simulink model "MODOSDESLISANTES"  (R2025a)
settings: Solver=VariableStepAuto  StartTime=0.0  StopTime=10.0  RelTol=1e-3
InitFcn:
  | % --- Código para el InitFcn ---
  | 
  | % Añadir la API al path (asegúrate que la ruta es correcta)
  | addpath('C:/RoboDK/Matlab/');
  | 
  | % Declarar las variables como globales
  | global RDK;
  | global ROBOT;
  | 
  | % Iniciar la conexión
  | RDK = Robolink();
  | 
  | % Obtener tu robot (CAMBIA 'MiRobot' por el nombre de tu robot)
  | ROBOT = RDK.Item('Fanuc CRX-5iA', RDK.ITEM_TYPE_ROBOT);
  | 
  | % Fallar si no se encuentra
  | if ~ROBOT.Valid()
  |     error('No se encontró el robot "MiRobot" en RoboDK.');
  | end
  | 
  | % Ajustar el modo de ejecución a SIMULATE
  | % Esto es necesario para que el streaming funcione bien.
  | RDK.setRunMode(RDK.RUNMODE_SIMULATE);
  | 
  | % Mover a una posición inicial de forma segura (opcional)
  | % ROBOT.MoveJ([0, -90, 0, -90, 0, 0]);
  | 
  | fprintf('RoboDK Conectado y listo para Simulink.\n');
  | % --- Fin del código InitFcn ---
libraries: robotmaniplib x1, robotsim3dlib x1, sim3dlib x1
settings Model: Creator=Sandro  LastModifiedBy=jaros

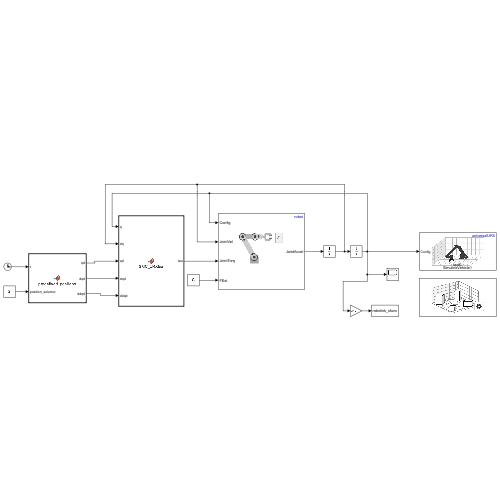
[thumbnail: Simulink's stored preview of the top-level diagram]
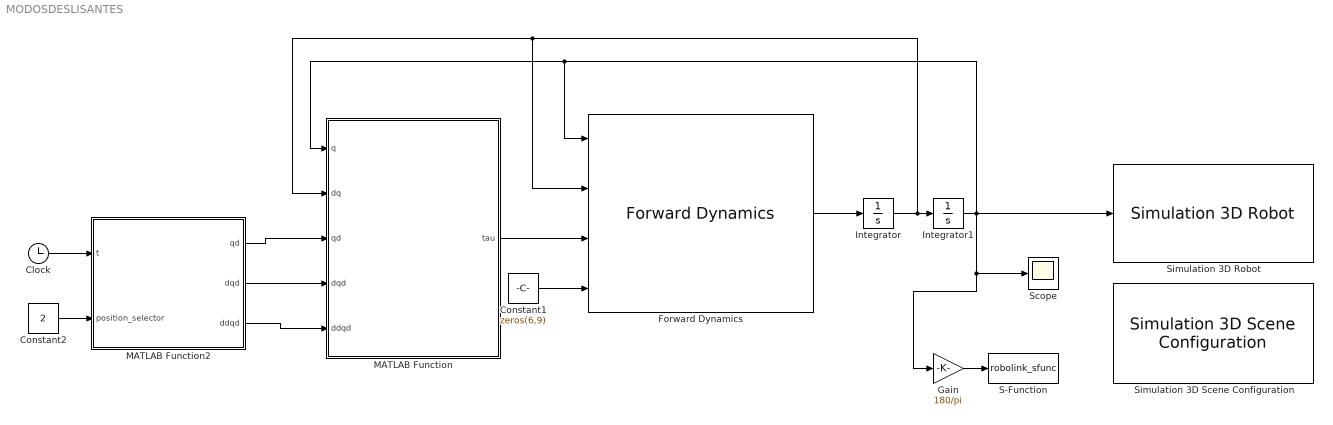
== system MODOSDESLISANTES ==
  Clock : Clock
  Constant1 : Constant  Value=zeros(6,9)
  Constant2 : Constant  Value=2
  Forward Dynamics : robotmaniplib/Forward Dynamics  RigidBodyTree=robot  SimulateUsing=Interpreted execution
  Gain : Gain  Gain=180/pi
  Integrator : Integrator
  Integrator1 : Integrator
  MATLAB Function : MATLAB Function  TreatAsAtomicUnit=on
  MATLAB Function2 : MATLAB Function  TreatAsAtomicUnit=on
  S-Function : S-Function  FunctionName=robolink_sfunc  SFunctionDeploymentMode=off  EnableBusSupport=off
  Scope : Scope
      settings: ActiveDisplayYMinimum=-2.2920470926945278  ActiveDisplayYMaximum=1.7511974378235475
  Simulation 3D Robot : robotsim3dlib/Simulation 3D Robot  actorInputType=Robot Library  RigidBodyTree=universalUR5  ActorName=SimulinkVehicle1  existActorChekBox=off  initialTrans=[0 0 0]  initialRot=[0 0 0]  initialConfig="[0  0  0  0  0  0]"  EndEffector=tool0  eeOffsetInpChekBox=off  eeTargetTrans=[0 0 0]  eeTargetRot=[0 0 0]  enableRegionGraspChekBox=off  regionGraspInpChekBox=off  eeTargTransDiff=[0.2 0.2 0.2]  eeTargRotDiff=[0 0 0]  enableVisualVisualization=on  enableCollisionVisualization=off  collisionGeomColor=[0 1 0]  collisionGeomTransp=0.1  inpConfEnbVal=on  inpGraspEnbVal=off  inpTransEnbVal=off  outConfEnbVal=off  outGraspEnbVal=off  outTransEnbVal=off  SampleTime=0.01  ActorType=SimulinkVehicle  ID=1  aMode=6  ActorTag=SimulinkVehicle1  Mesh=RigidBodyTree
  Simulation 3D Scene Configuration : sim3dlib/Simulation 3D Scene Configuration  Priority=0  ProjectFormat=Default Scenes  SceneDesc=Empty scene  ProjectName=C:\Program Files\MATLAB\R2025a\toolbox\shared\sim3d_projects\automotive_project_windows\UE\WindowsNoEditor\VehicleSimulation.exe  ScenePath=/Game/Maps/EmptyScene  EnableOpenDRIVE=off  vehTagList={'<empty>';'Custom';'Scene Origin';'SimulinkVehicle1'}  vehTag=Scene Origin  AttachedCameraRelativeTranslation=[0 0 0]  FreeCameraDefaultInitialTranslation=[-6, 0, 2]  AttachedCameraRelativeRotation=[0 0 0]  FreeCameraDefaultInitialRotation=[0, -15, 0]  ViewpointName=Custom  FreeCameraInitialTranslation=[0 0 0]  ViewpointTranslation=[0 0 0]  FreeCameraInitialRotation=[0 0 0]  ViewpointRotation=[0 0 0]  OpVisEn=off  Ts=0.02  EnableWindow=on  EnableRemoteAccess=off  EnableWeather=off  SunAzimuth=90  SunAltitude=40.0  EnableGeospatialSun=off  Latitude=0  Longitude=0  Date=2023-01-01  Time=10:30:00  GeoTimeZone=-5.0  SunDaylightSaving=off  wind=1  clouds=10  EnableVolumetricClouds=off  CloudCoverage=0  CloudAltitude=6  fog=0  rain=0  RaindropsEffect=off  SnowDensity=0  EnableGeospatial=off  TilesetSource=Earth terrain  UseTrueOrigin=off  OriginHeight=200  OriginLatitude=40.744652  OriginLongitude=-73.988864  MapStyle=Aerial  AdditionalAssetIDs=[]  UseAdvancedSunSky=off  SolarTime=11  TimeZone=-5  Day=21  Month=9  Year=2022  UseDaylightSavingTime=on  DSTStartDay=10  DSTStartMonth=3  DSTEndDay=3  DSTEndMonth=11  DSTSwitchHour=2  sensorTag=MainCamera1  sensorId=1  sensorName=MainCamera1  mountLoc=Origin  offsetFlag=off  tmountOffset=[0, 0, 0]  rmountOffset=[0, 0, 0]  HorizontalResolution=1280  VerticalResolution=720  HorizontalFOV=60  mountPoint=[0 0 0]  mountOrientation=[0 0 0]  aMode=6  ID=1  GeoTrigger=Inactive  ViewNameList={'Custom'}  ViewTranslationList={'[0 0 0]'}  ViewRotationList={'[0 0 0]'}
      settings: LibrarySourceBlock=robotsim3dlib/Simulation 3D Scene Configuration
  wires:
  Forward Dynamics/1 -> Integrator/1
  Integrator/1 -> MATLAB Function/2(dq), Forward Dynamics/2, Integrator1/1
  Integrator1/1 -> Simulation 3D Robot/1, Scope/1, Gain/1, Forward Dynamics/1, MATLAB Function/1(q)
  Constant1/1 -> Forward Dynamics/4
  MATLAB Function2/2(dqd) -> MATLAB Function/4(dqd)
  Constant2/1 -> MATLAB Function2/2(position_selector)
  MATLAB Function2/3(ddqd) -> MATLAB Function/5(ddqd)
  Clock/1 -> MATLAB Function2/1(t)
  MATLAB Function2/1(qd) -> MATLAB Function/3(qd)
  MATLAB Function/1(tau) -> Forward Dynamics/3
  Gain/1 -> S-Function/1

== matlab function MODOSDESLISANTES/MATLAB Function ==
  data: q input; dq input; tau output; qd input; dqd input; ddqd input
function tau = SMC_CRX5ia(q, dq, qd, dqd, ddqd)
% Control por Modos Deslizantes para Fanuc CRX-5ia
% Parámetros definidos internamente - Sin estructura
%
% Inputs:
%   q, dq      : Estados actuales [6x1] (rad, rad/s)
%   qd, dqd, ddqd: Trayectoria deseada [6x1]
%
% Output:
%   tau        : Vector de torque [6x1] (Nm)

%#codegen
tau = zeros(6,1); % Especificar tamaño de salida

% =========================================================================
% PARÁMETROS DEFINIDOS INTERNAMENTE (Basados en URDF del CRX-5ia)
% =========================================================================

% 1. MATRIZ DE INERCIA ESTIMADA [kg·m²]
M_hat = diag([2.5, 1.8, 1.2, 0.8, 0.5, 0.3]);

% 2. MATRIZ DE CORIOLIS ESTIMADA
C_hat = zeros(6,6); % Simplificación inicial

% 3. VECTOR DE GRAVEDAD [Nm]
g_hat = [0; 12.5; 8.8; 0; 2.9; 0.3];

% 4. MATRIZ DE GANANCIAS DE SUPERFICIE DESLIZANTE
Lambda = diag([8, 8, 10, 12, 15, 15]);

% 5. MATRIZ DE GANANCIAS DISCONTINUAS
K = diag([25, 20, 15, 10, 8, 5]);

% 6. PARÁMETRO DE ROBUSTEZ
eta = 3;

% 7. CONFIGURACIÓN ANTI-CHATTERING
use_saturation = true;
phi = 0.15;

% 8. LÍMITES ARTICULARES (del URDF)
q_min = [-2*pi, -2*pi, -pi, -2*pi, -2*pi, -2*pi]';
q_max = [2*pi, 2*pi, pi, 2*pi, 2*pi, 2*pi]';
dq_max = [3.15, 3.15, 3.15, 3.2, 3.2, 3.2]';

% =========================================================================
% ALGORITMO DE CONTROL POR MODOS DESLIZANTES
% =========================================================================

% Verificación de límites articulares
q = clamp(q, q_min, q_max);
dq = clamp(dq, -dq_max, dq_max);

% Cálculo de errores
q_tilde = q - qd;
dq_tilde = dq - dqd;

% Velocidad y aceleración de referencia
dq_r = dqd - Lambda * q_tilde;
ddq_r = ddqd - Lambda * dq_tilde;

% Superficie deslizante
s = dq - dq_r;

% Control equivalente
tau_eq = M_hat * ddq_r + C_hat * dq_r + g_hat;

% Término robusto (con saturación para reducir chattering)
if use_saturation
    s_robust = saturation(s, phi);
else
    s_robust = sign(s);
end

% Ley de control final
tau = tau_eq - K * s_robust - eta * s;

% Limitar torque de salida para protección
tau_max = [100, 80, 60, 40, 30, 20]'; % [Nm] límites conservadores
tau = clamp(tau, -tau_max, tau_max);

end

% =========================================================================
% FUNCIONES AUXILIARES
% =========================================================================

function s_sat = saturation(s, phi)
% Función de saturación para reducir chattering
    s_sat = zeros(size(s));
    for i = 1:length(s)
        if abs(s(i)) > phi
            s_sat(i) = sign(s(i));
        else
            s_sat(i) = s(i) / phi;
        end
    end
end

function y = clamp(x, min_val, max_val)
% Función de limitación de valores
    y = min(max(x, min_val), max_val);
end

== matlab function MODOSDESLISANTES/MATLAB Function2 ==
  data: qd output; t input; position_selector input; dqd output; ddqd output
function [qd, dqd, ddqd] = predefined_positions(t, position_selector)
% Posiciones predefinidas para el CRX-5ia
%
% position_selector:
%   1: Home (todo ceros)
%   2: Configuración extendida
%   3: Configuración recogida
%   4: Posición de trabajo
%   5: Personalizada (puedes agregar más)

    % Definir posiciones preestablecidas [rad]
    switch position_selector
        case 1 % HOME
            desired_q = [0, 0, 0, 0, 0, 0]';
        case 2 % EXTENDIDO
            desired_q = [0, -pi/2, pi/2, 0, 0, 0]';
        case 3 % RECOGIDO  
            desired_q = [0, -pi/4, pi/4, 0, 0, 0]';
        case 4 % TRABAJO
            desired_q = [pi/6, -pi/3, pi/3, 0, pi/4, 0]';
        case 5 % PERSONALIZADA 1
            desired_q = [pi/4, -pi/6, pi/6, pi/8, 0, 0]';
        otherwise % HOME por defecto
            desired_q = [0, 0, 0, 0, 0, 0]';
    end
    
    % Usar transición suave desde la posición actual
    transition_time = 3.0; % 3 segundos para llegar
    
    if t < transition_time
        % Transición suave
        s = t / transition_time;
        qd = desired_q * (3*s^2 - 2*s^3); % De [0,0,0...] a desired_q
        dqd = desired_q * (6*s - 6*s^2) / transition_time;
        ddqd = desired_q * (6 - 12*s) / (transition_time^2);
    else
        % Mantener posición deseada
        qd = desired_q;
        dqd = zeros(6,1);
        ddqd = zeros(6,1);
    end
    
end
